simulink model "TrayectoriaObstaculos"  (R2023b)
settings: Solver=FixedStepDiscrete  StartTime=0.0  StopTime=150  FixedStep=0.01  RelTol=1e-3  EnableMultiTasking=on
model workspace (MAT data in the model file):
  d = 0.22
libraries: slpidlib x1
settings Model: ExtModeTrigDuration=2  Creator=Andrés  LastModifiedBy=Andrés
settings SolverCC: AutoInsertRateTranBlk=on
settings OptimizationCC: EnhancedBackFolding=on  PassReuseOutputArgsAs=Individual arguments  ZeroExternalMemoryAtStartup=off  ZeroInternalMemoryAtStartup=off  MaxStackSize=64  OptimizeBlockOrder=speed  DifferentSizesBufferReuse=on  EfficientTunableParamExpr=on
settings DebuggingCC: ParameterTunabilityLossMsg=error
settings HardwareCC: ProdBitPerInt=16  ProdBitPerPointer=16  ProdBitPerSizeT=16  ProdBitPerPtrDiffT=16  ProdLargestAtomicFloat=None  ProdWordSize=8  ProdHWDeviceType=Atmel->AVR  UseEmbeddedCoderFeatures=off  UseSimulinkCoderFeatures=off
settings SFSimCC: MATLABDynamicMemAlloc=off
settings RTWCC: Description=Embedded Coder  SystemTargetFile=ert.tlc  HardwareBoard=Arduino Mega 2560  TemplateMakefile=ert_default_tmf  Toolchain=Arduino AVR  BuildConfiguration=Faster Runs
settings CodeAppCC: ForceParamTrailComments=on  IgnoreCustomStorageClasses=off  OperatorAnnotations=on  SimulinkDataObjDesc=on  SFDataObjDesc=on  InsertBlockDesc=on
settings ERTTargetCC: SupportContinuousTime=on  SupportNonInlinedSFcns=on  SupportVariableSizeSignals=on  ExtModeTransport=3  ExtModeStaticAlloc=on  ExtModeAutomaticAllocSize=off  ExtModeStaticAllocSize=2048  ExtModeMexFile=ext_xcp  ExtModeIntrfLevel=Level2 - Open

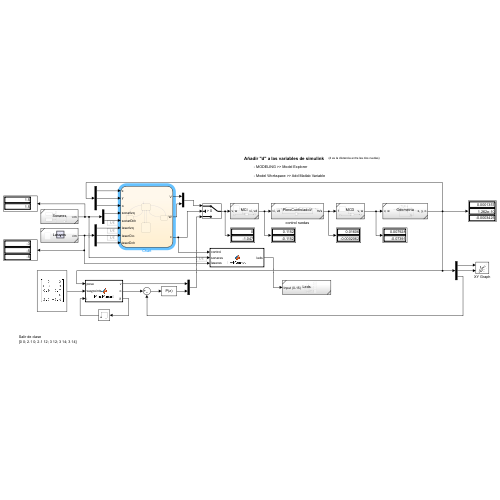
[thumbnail: Simulink's stored preview of the top-level diagram]
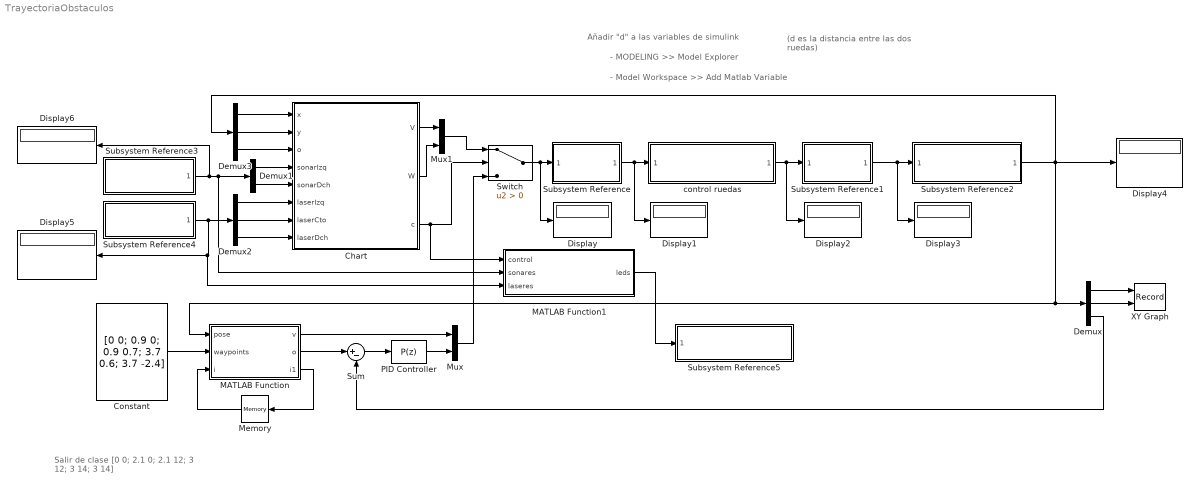
== system TrayectoriaObstaculos ==
  note: Salir de clase
      | [0 0; 2.1 0; 2.1 12; 3 12; 3 14; 3 14]
  note: (d es la distancia entre las dos ruedas)
  note: - Model Workspace >> Add Matlab Variable
  note: - MODELING >> Model Explorer
  note: Añadir "d" a las variables de simulink
  Chart : Stateflow chart  TreatAsAtomicUnit=on
  Constant : Constant  Value=[0 0; 0.9 0; 0.9 0.7; 3.7 0.6; 3.7 -2.4]
  Demux : Demux  Outputs=3
  Demux1 : Demux  Outputs=2
  Demux2 : Demux  Outputs=3
  Demux3 : Demux  Outputs=3
  Display{,1..6} (7 alike) : Display
  MATLAB Function : MATLAB Function  TreatAsAtomicUnit=on
  MATLAB Function1 : MATLAB Function  TreatAsAtomicUnit=on
  Memory : Memory
  Mux : Mux  Inputs=2
  Mux1 : Mux  Inputs=2
  PID Controller : slpidlib/PID Controller  Controller=P  Form=Parallel  TimeDomain=Discrete-time  UseExternalTs=off  SampleTime=-1  IntegratorMethod=Forward Euler  FilterMethod=Forward Euler  ControllerParametersSource=internal  P=1.50579034682725  I=1  UseKiTs=off  D=0  N=100  UseFilter=on  TunerSelectOption=Transfer Function Based (PID Tuner App)  InitialConditionSource=internal  InitialConditionForIntegrator=0  InitialConditionForFilter=0  DifferentiatorICPrevScaledInput=0  ExternalReset=none  TrackingMode=off  Kt=1  LimitOutput=off  SatLimitsSource=internal  UpperSaturationLimit=inf  LowerSaturationLimit=-inf  LinearizeAsGain=on  AntiWindupMode=none  Kb=1  LimitIntegrator=off  UpperIntegratorSaturationLimit=inf  LowerIntegratorSaturationLimit=-inf  POutMin=[]  POutMax=[]  IOutMin=[]  IOutMax=[]  DOutMin=[]  DOutMax=[]  NOutMin=[]  NOutMax=[]  SumOutMin=[]  SumOutMax=[]  SaturationOutMin=[]  SaturationOutMax=[]  PParamMin=[]  PParamMax=[]  IParamMin=[]  IParamMax=[]  DParamMin=[]  DParamMax=[]  NParamMin=[]  NParamMax=[]  KbParamMin=[]  KbParamMax=[]  KtParamMin=[]  KtParamMax=[]  KbOutMin=[]  KbOutMax=[]  KtOutMin=[]  KtOutMax=[]  IntegratorOutMin=[]  IntegratorOutMax=[]  FilterOutMin=[]  FilterOutMax=[]  SumI1OutMin=[]  SumI1OutMax=[]  SumI2OutMin=[]  SumI2OutMax=[]  SumI3OutMin=[]  SumI3OutMax=[]  SumI4OutMin=[]  SumI4OutMax=[]  SumDOutMin=[]  SumDOutMax=[]  DifferentiatorOutMin=[]  DifferentiatorOutMax=[]  FilterDiffOutCoefMin=[]  FilterDiffOutCoefMax=[]  ReciprocalOutMin=[]  ReciprocalOutMax=[]  SumDenOutMin=[]  SumDenOutMax=[]  SumNumOutMin=[]  SumNumOutMax=[]  DivideOutMin=[]  DivideOutMax=[]  UdiffTsProdOutMin=[]  UdiffTsProdOutMax=[]  NTsProdOutMin=[]  NTsProdOutMax=[]  UintegralTsProdOutMin=[]  UintegralTsProdOutMax=[]  UngainTsProdOutMin=[]  UngainTsProdOutMax=[]  ClampingZeroOutDataTypeStr=Inherit: Inherit via back propagation  ClampingZeroOutMin=[]  ClampingZeroOutMax=[]  FilterDenConstantOutDataTypeStr=Inherit: Inherit via back propagation  FilterDenConstantOutMin=[]  FilterDenConstantOutMax=[]  PCopyOutDataTypeStr=Inherit: Inherit via back propagation  PCopyOutMin=[]  PCopyOutMax=[]  NCopyOutDataTypeStr=Inherit: Inherit via back propagation  NCopyOutMin=[]  NCopyOutMax=[]  IntegratorContinuousStateAttributes=''  IntegratorStateMustResolveToSignalObject=off  IntegratorRTWStateStorageClass=Auto  FilterContinuousStateAttributes=''  FilterStateMustResolveToSignalObject=off  FilterRTWStateStorageClass=Auto  ParallelPVariant=InternalParameters  IdealPVariant=Disabled  IVariant=Disabled  DVariant=Disabled  IntegratorVariant=Disabled  SatVariant=Disabled  AWVariant=Disabled  PCopyVariant=Disabled  TRVariant=Disabled  FdbkBlocksVariant=Forward  IdealPFdbkVariant=Disabled  SatFdbkVariant=Disabled  DerivativeFilterVariant=Disabled  NVariant=Disabled  NCopyVariant=Disabled_SignalSpec  FilterICVariant=Disabled  IntegratorICVariant=Disabled  ExternalResetVariant=Disabled  TRSumVariant=Passthrough  SumFdbkVariant=Disabled  SumVariant=Passthrough_P  TsampFilterVariant=InternalTs  TsampNgainVariant=Passthrough  TsampIntegralVariant=Disabled_SignalSpec  ExternalSaturationOutDataTypeStr=Inherit: Same as second input
  Subsystem Reference : Subsystem  ReferencedSubsystem=MCI
  Subsystem Reference1 : Subsystem  ReferencedSubsystem=MCD
  Subsystem Reference2 : Subsystem  ReferencedSubsystem=Odometria
  Subsystem Reference3 : Subsystem  ReferencedSubsystem=Sonares
  Subsystem Reference4 : Subsystem  ReferencedSubsystem=Laseres
  Subsystem Reference5 : Subsystem  ReferencedSubsystem=Leds
  Sum : Sum  Inputs=|+-
  Switch : Switch  Criteria=u2 > Threshold  SaturateOnIntegerOverflow=off  InputSameDT=off
  XY Graph : Record  FileSettingsInternal="{\"entries\":[{\"content\":{\"excelSettings\":{\"content\":{},\"type\":\"Streamout.ExcelSettings\"}},\"type\":\"Streamout.FileSettingStorage\",\"uuid\":\"\"}],\"packageUris\":[\"http:\\/\\/schema.mathworks.com\\/mf0\\/streamout_blocks\\/R2020a\"],\"version\":\"1.0\"}"  Layout=[1 1]  SignalsInternal="{\"entries\":[{\"content\":{\"signals\":[{\"content\":{\"blockPath\":[],\"dimensions\":[1],\"domain\":\"\",\"lineColor\":\"#a2142f\",\"plots\":[ 1 ],\"port\":1,\"sid\":[\"\"],\"signalID\":1,\"signalName\":\"Demux:1\"},\"type\":\"RecordBlkView.Signal\",\"uuid\":\"\"},{\"content\":{\"blockPath\":[],\"dimensions\":[1],\"domain\":\"\",\"lineColor\":\"#139fff\",\"plots\":[ 1 ],\"port\":2,\"sid\":[\"\"],\"signalID\":2,\"signalName\":\"Demux:2\"},\"type\":\"RecordBlkView.Signal\",\"uuid\":\"\"}]},\"type\":\"RecordBlkView.InputSignals\",\"uuid\":\"\"}],\"packageUris\":[\"http:\\/\\/schema.mathworks.com\\/mf0\\/streamout_blocks\\/R2020a\"],\"version\":\"1.0\"}"  VisualizationBindings="{\"xyplotplugin\":{\"info\":[{\"series\":[{\"bindingParametersList\":[{\"parameter\":\"X-Axis\",\"signalID\":1,\"signalName\":\"Demux:1\"},{\"parameter\":\"Y-Axis\",\"signalID\":2,\"signalName\":\"Demux:2\"}],\"seriesID\":0}],\"subplotID\":1}]}}"  CompatibilityTag=XY
  control ruedas : Subsystem  ReferencedSubsystem=PieroControladoV
  wires:
  control ruedas/1 -> Display2/1, Subsystem Reference1/1
  Subsystem Reference1/1 -> Display3/1, Subsystem Reference2/1
  Subsystem Reference/1 -> Display1/1, control ruedas/1
  Demux/2 -> XY Graph/2
  Subsystem Reference2/1 -> Demux3/1, Demux/1, MATLAB Function/1(pose), Display4/1
  Demux/1 -> XY Graph/1
  Demux/3 -> Sum/2
  Sum/1 -> PID Controller/1
  PID Controller/1 -> Mux/2
  MATLAB Function/1(v) -> Mux/1
  MATLAB Function/2(o) -> Sum/1
  MATLAB Function/3(i1) -> Memory/1
  Memory/1 -> MATLAB Function/3(i)
  Constant/1 -> MATLAB Function/2(waypoints)
  Switch/1 -> Display/1, Subsystem Reference/1
  Mux/1 -> Switch/3
  Subsystem Reference3/1 -> Display6/1, MATLAB Function1/2(sonares), Demux1/1
  Subsystem Reference4/1 -> Demux2/1, MATLAB Function1/3(laseres), Display5/1
  Demux2/3 -> Chart/8(laserDch)
  Demux2/2 -> Chart/7(laserCto)
  Demux2/1 -> Chart/6(laserIzq)
  Demux1/2 -> Chart/5(sonarDch)
  Demux1/1 -> Chart/4(sonarIzq)
  Demux3/1 -> Chart/1(x)
  Demux3/2 -> Chart/2(y)
  Demux3/3 -> Chart/3(o)
  Chart/3(c) -> MATLAB Function1/1(control), Switch/2
  Chart/1(V) -> Mux1/1
  Chart/2(W) -> Mux1/2
  Mux1/1 -> Switch/1
  MATLAB Function1/1(leds) -> Subsystem Reference5/1

== matlab function TrayectoriaObstaculos/MATLAB Function1 ==
  data: control input; leds output; sonares input; laseres input
function leds = LedControl(control, sonares, laseres)
% Función para controlar los leds. Salida entero del 1-15
    % 1:  Azul
    % 2:  Verde
    % 3:  Cyan
    % 4:  Rojo
    % 5:  Rosa
    % 6:  Amarillo
    % 7:  Blanco
    % 8:  -----------------
    % 9:  Azul Intermitente
    % 10: Verde Intermitente
    % 11: Cyan Intermitente
    % 12: Rojo Intermitente
    % 13: Rosa Intermitente
    % 14: Amarillo Intermitente
    % 15: Blanco Intermitente

sonarIzq = sonares(1);
sonarDch = sonares(2);

laserIzq = laseres(1);
laserCto = laseres(2);
laserDch = laseres(3);
    
leds = 2;

if(control == 1)
    leds = 12;    
end

== matlab function TrayectoriaObstaculos/MATLAB Function ==
  data: pose input; v output size=1; waypoints input; i input; o output size=1; i1 output size=1
function [v, o, i1] = PurePursuit(pose, waypoints, i)

% Margen de distancia
LA = 0.20;

%Inicializamos variables
v = 0.205;
o = 0;
if(isempty(i) || i < 1)
    i = 1;
end

% Extraemos la posición
x = pose(1);
y = pose(2);

if(length(waypoints) >= i)
    distancia = sqrt((waypoints(i,1)-x)^2 + (waypoints(i,2)-y)^2);

    if(distancia > LA)
        o = atan2(waypoints(i,2)-y, waypoints(i,1)-x);
        v = 0.205;
    else
        i = i+1;
    end    
else
    o = 0;
    v = 0;
end

i1 = i;

== stateflow chart TrayectoriaObstaculos/Chart ==
  state SinObstaculos
    V = 0;
    W = 0;
    c = 0;
  state ObstaculoIzq
    V = 0.1;
    W = -pi/4;
    c = 1;
  state ObstaculoDch
    V = 0.1;
    W = pi/4;
    c = 1;
  state ObstaculoFrente
    V = 0;
    c = 1;
    if laserDch < laserIzq
    W = pi/3;
    else
    W = -pi/3;
    end
  (default) -> SinObstaculos
  SinObstaculos -> ObstaculoDch [order 3] : [laserDch < 25]
  SinObstaculos -> ObstaculoIzq [order 2] : [laserIzq < 25]
  ObstaculoIzq -> SinObstaculos : after(1, sec)
  SinObstaculos -> ObstaculoFrente [order 1] : [laserCto < 15]
  ObstaculoFrente -> SinObstaculos : after(1.5, sec)
  ObstaculoDch -> SinObstaculos : after(1, sec)
  data: x input; y input; o input; sonarIzq input; sonarDch input; laserIzq input; laserCto input; laserDch input; V output; W output; c output
